simulink model "controle_simples"  (R2016a)
settings: Solver=ode45  StartTime=0.0  StopTime=10.0  RelTol=1e-3
libraries: simulink x1
settings Model: Creator=Administrator  LastModifiedBy=vmaraccini-personal
settings DataIOCC: LimitDataPoints=on  SaveFormat=Array
settings HardwareCC: ProdBitPerPointer=32  ProdLargestAtomicFloat=None  ProdIntDivRoundTo=Undefined  ProdEndianess=Unspecified  ProdWordSize=32  ProdHWDeviceType=32-bit Generic
settings ModelReferenceCC: ModelReferenceNumInstancesAllowed=Single  PropagateSignalLabelsOutOfModel=off
settings ConfigComp: CovModelRefEnable=Off

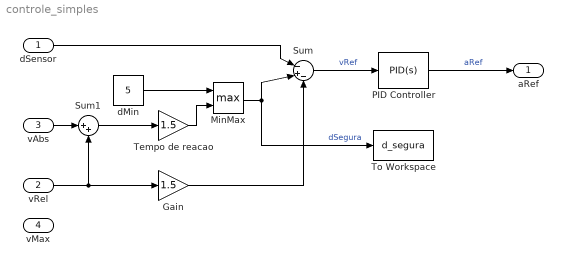
== system controle_simples ==
  dSensor : Inport
  vRel : Inport  Port=2
  vAbs : Inport  Port=3
  vMax : Inport  Port=4
  Gain : Gain  Gain=1.5
  MinMax : MinMax  Function=max  Inputs=2  OutMin=10
  PID Controller : simulink/Continuous/PID Controller  Controller=PID  TimeDomain=Continuous-time  SampleTime=-1  IntegratorMethod=Forward Euler  FilterMethod=Forward Euler  Form=Parallel  UseFilter=on  ControllerParametersSource=internal  P=-3.87280472505017  I=-1.31628778505579  D=-0.931121700721534  N=1.02327765217534  InitialConditionSource=internal  InitialConditionForIntegrator=0  InitialConditionForFilter=0  ExternalReset=none  LimitOutput=on  UpperSaturationLimit=100  LowerSaturationLimit=-100  LinearizeAsGain=on  AntiWindupMode=none  Kb=1  TrackingMode=off  Kt=1  PParamMin=[]  PParamMax=[]  IParamMin=[]  IParamMax=[]  DParamMin=[]  DParamMax=[]  NParamMin=[]  NParamMax=[]  KbParamMin=[]  KbParamMax=[]  KtParamMin=[]  KtParamMax=[]  POutMin=[]  POutMax=[]  IOutMin=[]  IOutMax=[]  DOutMin=[]  DOutMax=[]  NOutMin=[]  NOutMax=[]  KbOutMin=[]  KbOutMax=[]  KtOutMin=[]  KtOutMax=[]  IntegratorOutMin=[]  IntegratorOutMax=[]  FilterOutMin=[]  FilterOutMax=[]  SumOutMin=[]  SumOutMax=[]  SumI1OutMin=[]  SumI1OutMax=[]  SumI2OutMin=[]  SumI2OutMax=[]  SumI3OutMin=[]  SumI3OutMax=[]  SumDOutMin=[]  SumDOutMax=[]  SaturationOutMin=[]  SaturationOutMax=[]  IntegratorContinuousStateAttributes=''  IntegratorStateMustResolveToSignalObject=off  IntegratorRTWStateStorageClass=Auto  FilterContinuousStateAttributes=''  FilterStateMustResolveToSignalObject=off  FilterRTWStateStorageClass=Auto  DifferentiatorICPrevScaledInput=0  DifferentiatorOutMin=[]  DifferentiatorOutMax=[]
  Sum : Sum  Inputs=|-+-
  Sum1 : Sum  Inputs=|++
  Tempo de reacao : Gain  Gain=1.5
  To Workspace : ToWorkspace  VariableName=d_segura  SampleTime=-1
      settings: Save2DSignal=2-D array (concatenate along first dimension)
  dMin : Constant  Value=5
  aRef : Outport
  wires:
  dSensor/1 -> Sum/1
  Sum/1 -> PID Controller/1  "vRef"
  vRel/1 -> Gain/1, Sum1/2
  MinMax/1 -> To Workspace/1, Sum/2  "dSegura"
  Tempo de reacao/1 -> MinMax/2
  dMin/1 -> MinMax/1
  Sum1/1 -> Tempo de reacao/1
  vAbs/1 -> Sum1/1
  Gain/1 -> Sum/3
  PID Controller/1 -> aRef/1  "aRef"
